simulink model "bot_m"  (R2023b)
settings: Solver=FixedStepAuto  StartTime=0.0  StopTime=SIM_TIME  FixedStep=STEP_SIZE  RelTol=1e-3
values from neighbouring files (symbols this model uses):
  dtheta0 = 0    [bot.m]
  g = 9.82    [bot.m]
  I = 1/3*m*L^2    (= 0.036)    [bot.m]    (also in motor.m = 6e-05)
  m = 0.3    [bot.m]
  STEP_SIZE = 1e-3    (= 0.001)    [bot.m]
  theta0 = deg2rad(15)    [bot.m]
settings Model: Creator=farfar  LastModifiedBy=farfar
settings DataIOCC: ReturnWorkspaceOutputs=off

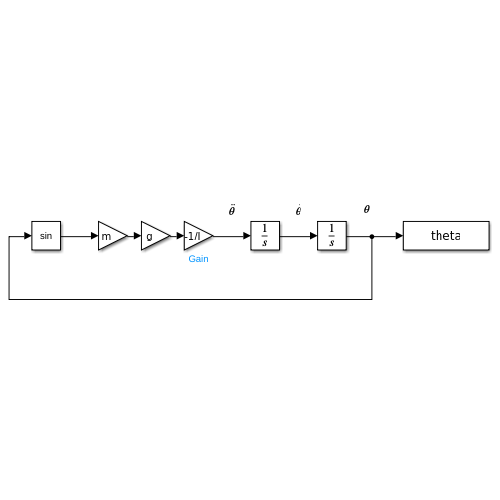
[thumbnail: Simulink's stored preview of the top-level diagram]
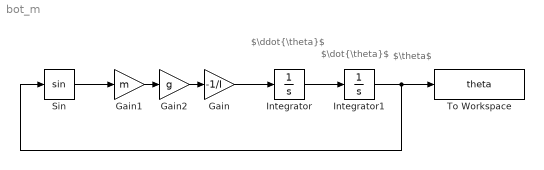
== system bot_m ==
  note: $\theta$
  note: $\dot{\theta}$
  note: $\ddot{\theta}$
  Gain : Gain  Gain=-1/I
  Gain1 : Gain  Gain=m
  Gain2 : Gain  Gain=g
  Integrator : Integrator  InitialCondition=dtheta0  ContinuousStateAttributes='dtheta'
  Integrator1 : Integrator  InitialCondition=theta0  ContinuousStateAttributes='theta'
  Sin : Trigonometry
  To Workspace : ToWorkspace  VariableName=theta  SampleTime=STEP_SIZE
  wires:
  Gain1/1 -> Gain2/1
  Gain2/1 -> Gain/1
  Sin/1 -> Gain1/1
  Gain/1 -> Integrator/1
  Integrator/1 -> Integrator1/1
  Integrator1/1 -> To Workspace/1, Sin/1
